simulink model "DataType"  (R2021b)
settings: Solver=VariableStepAuto  StartTime=0.0  StopTime=10.0  RelTol=1e-3
undefined symbols (not defined in the file): DiscIntNeverNeededParam, magnitude, Newton, Raphson
libraries: simulink x4, slpidlib x1
settings Model: Creator=user  LastModifiedBy=cemery

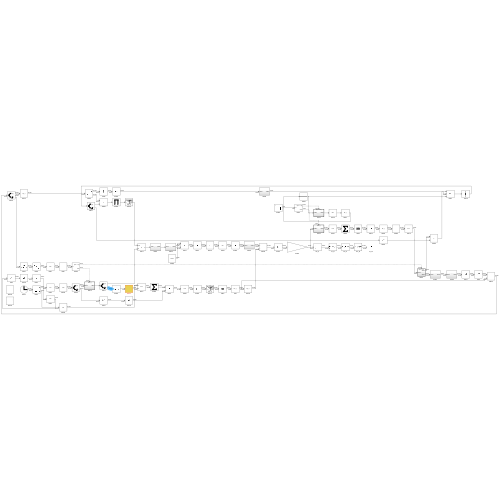
[thumbnail: Simulink's stored preview of the top-level diagram]
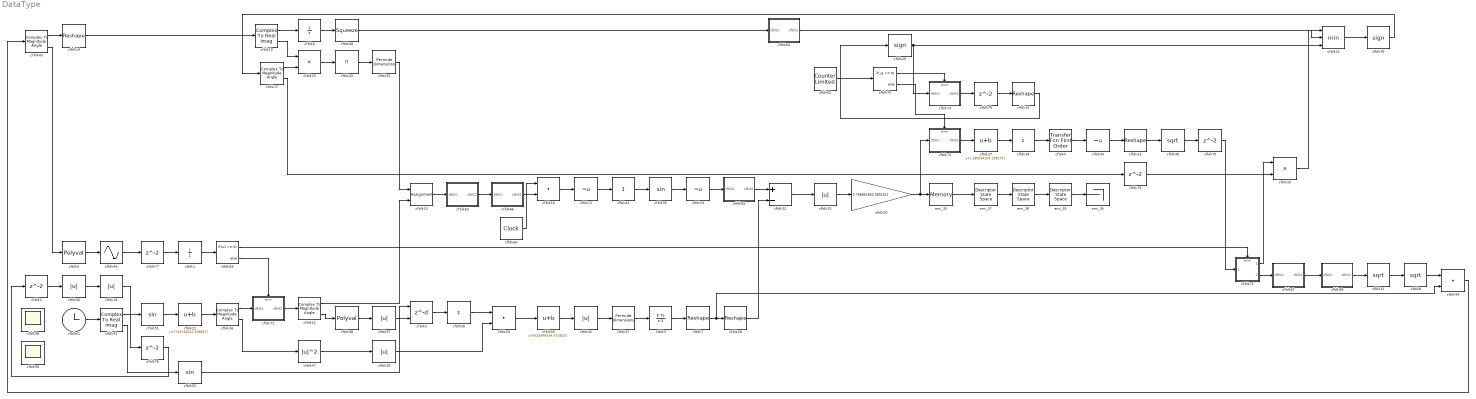
== system DataType ==
  cfblk1 : UnitDelay  HasFrameUpgradeWarning=on
  cfblk{10,18,30,42,56..57} (6 alike) : Abs
  cfblk11 : UnaryMinus
  cfblk{12,17,36,43} (4 alike) : ComplexToMagnitudeAngle
  cfblk13 : Assignment  DiagnosticForDimensions=Warning  IndexOptions=Index vector (dialog)  Indices=1  OutputSizes=1
  cfblk{7,14..15,23,28} (5 alike) : Reshape
  cfblk16 : DotProduct  InputSameDT=on  OutDataTypeStr=Inherit: Inherit via internal rule
  cfblk19 : ComplexToRealImag
  cfblk{2,75..79} (6 alike) : Delay  SampleTime=1
  cfblk20 : Gain  Gain=[-758951851.585151]
  cfblk21 : MinMax  Inputs=3
  cfblk22 : Bias  Bias=[749742041.378697]
  cfblk24 : simulink/Math Operations/Slider Gain  gain=1  low=0  high=2
  cfblk25 : Product
  cfblk26 : Sum  Inputs=+
  cfblk27 : Bias  Bias=[-185034104.199175]
  cfblk29 : Signum
  cfblk3 : Delay  DelayLengthSource=Input port  SampleTime=1
      settings: InputPortMap=u0,p1
  cfblk31 : Sqrt  SaturateOnIntegerOverflow=on
  cfblk32 : Sum  Inputs=+-
  cfblk33 : Product
  cfblk34 : UnaryMinus
  cfblk35 : Trigonometry
  cfblk37 : PermuteDimensions
  cfblk38 : Polyval  Coefs=[ +2.081618890e-019, -1.441693666e-014, +4.719686976e-010, -8.536869453e-006, +1.621573104e-001, -8.087801117e+001 ]
  cfblk39 : Sum  Inputs=+
  cfblk4 : simulink/Discrete/Transfer Fcn First Order  PoleZ=0.95  ICPrevOutput=0.0  DoSatur=off
  cfblk40 : Sqrt  SaturateOnIntegerOverflow=on
  cfblk41 : ComplexToRealImag
  cfblk44 : DotProduct  InputSameDT=on  OutDataTypeStr=Inherit: Inherit via internal rule
  cfblk45 : Product  Inputs=*
  cfblk46 : Sin  TimeSource=Use external signal  SampleTime=0
  cfblk47 : Math  Operator=magnitude^2  SaturateOnIntegerOverflow=on
  cfblk48 : Squeeze
  cfblk49 : Signum
  cfblk5 : DiscreteIntegrator  ICPrevOutput=DiscIntNeverNeededParam  ICPrevScaledInput=DiscIntNeverNeededParam
  cfblk50 : Bias  Bias=[622648534.571803]
  cfblk51 : Trigonometry
  cfblk52 : PermuteDimensions
  cfblk53 : DotProduct  InputSameDT=on  OutDataTypeStr=Inherit: Inherit via internal rule
  cfblk54 : UnaryMinus
  cfblk55 : Trigonometry
  cfblk58 : Scope
      settings: Floating=on
  cfblk59 : Scope
      settings: Floating=on
  cfblk6 : UnitDelay  HasFrameUpgradeWarning=on
  cfblk60 : DigitalClock
  cfblk61 : Clock
  cfblk62 : simulink/Sources/Counter Limited  uplimit=[209.000000]  tsamp=-1
  cfblk63 : Subsystem
  cfblk64 : Subsystem
  cfblk65 : Subsystem
  cfblk66 : Subsystem
  cfblk67 : Subsystem
  cfblk68 : Subsystem
  cfblk69 : If  IfExpression=u1 >= 0  SampleTime=1
  cfblk70 : If  IfExpression=u1 >= 0  SampleTime=1
  cfblk71 : Subsystem  TreatAsAtomicUnit=on
  cfblk72 : Subsystem  TreatAsAtomicUnit=on
  cfblk73 : Subsystem  TreatAsAtomicUnit=on
  cfblk74 : Subsystem  TreatAsAtomicUnit=on
  cfblk8 : Sqrt  SaturateOnIntegerOverflow=on
  cfblk9 : Polyval  Coefs=[ +2.081618890e-019, -1.441693666e-014, +4.719686976e-010, -8.536869453e-006, +1.621573104e-001, -8.087801117e+001 ]
  emi_35 : Memory
  emi_36 : Terminator
  emi_37 : DescriptorStateSpace
  emi_38 : DescriptorStateSpace
  emi_39 : DescriptorStateSpace
  wires:
  cfblk38/1 -> cfblk57/1
  cfblk52/1 -> cfblk13/1
  cfblk28/1 -> cfblk32/2
  cfblk74/1(cfblk2) -> cfblk27/1
  cfblk18/1 -> cfblk78/1
  cfblk73/1(cfblk2) -> cfblk79/1
  cfblk30/1 -> cfblk53/2
  cfblk70/2 -> cfblk74/Action
  emi_39/1 -> emi_36/1
  cfblk78/1 -> cfblk2/1
  cfblk26/1 -> cfblk53/1
  cfblk41/2 -> cfblk55/1
  cfblk61/1 -> cfblk41/1
  emi_38/1 -> emi_39/1
  cfblk1/1 -> cfblk69/1
  emi_37/1 -> emi_38/1
  cfblk19/2 -> cfblk25/1
  cfblk55/1 -> cfblk3/1
  cfblk46/1 -> cfblk77/1
  emi_35/1 -> emi_37/1
  cfblk9/1 -> cfblk46/1
  cfblk37/1 -> cfblk5/1
  cfblk12/2 -> cfblk38/1
  cfblk79/1 -> cfblk15/1
  cfblk77/1 -> cfblk1/1
  cfblk6/1 -> cfblk48/1
  cfblk4/1 -> cfblk34/1
  cfblk47/1 -> cfblk30/1
  cfblk76/1 -> cfblk33/2
  cfblk67/1(cfblk2) -> cfblk68/1(cfblk1)
  cfblk17/2 -> cfblk76/1
  cfblk49/1 -> cfblk17/1
  cfblk54/1 -> cfblk65/1(cfblk1)
  cfblk75/1 -> cfblk71/1(cfblk1)
  cfblk40/1 -> cfblk75/1
  cfblk25/1 -> cfblk45/1
  cfblk70/1 -> cfblk73/Action
  cfblk57/1 -> cfblk3/2
  cfblk69/2 -> cfblk72/Action
  cfblk69/1 -> cfblk71/Action
  cfblk19/1 -> cfblk6/1
  cfblk64/1(cfblk2) -> cfblk21/2
  cfblk51/1 -> cfblk22/1
  cfblk17/1 -> cfblk25/2
  cfblk71/1(cfblk2) -> cfblk33/1
  cfblk62/1 -> cfblk70/1
  cfblk32/1 -> cfblk10/1
  cfblk22/1 -> cfblk36/1
  cfblk21/1 -> cfblk49/1
  cfblk71/2(cfblk4) -> cfblk67/1(cfblk1)
  cfblk33/1 -> cfblk21/1
  cfblk2/1 -> cfblk56/1
  cfblk68/1(cfblk2) -> cfblk31/1
  cfblk36/2 -> cfblk47/1
  cfblk12/1 -> cfblk13/2
  cfblk14/1 -> cfblk19/1
  cfblk50/1 -> cfblk42/1
  cfblk66/1(cfblk2) -> cfblk16/2
  cfblk36/1 -> cfblk72/1(cfblk1)
  cfblk3/1 -> cfblk26/1
  cfblk16/1 -> cfblk11/1
  cfblk53/1 -> cfblk50/1
  cfblk41/1 -> cfblk51/1
  cfblk45/1 -> cfblk52/1
  cfblk27/1 -> cfblk39/1
  cfblk60/1 -> cfblk16/1
  cfblk15/1 -> cfblk29/1
  cfblk10/1 -> cfblk20/1
  cfblk11/1 -> cfblk24/1
  cfblk44/1 -> cfblk43/1
  cfblk34/1 -> cfblk23/1
  cfblk8/1 -> cfblk44/1
  cfblk63/1(cfblk2) -> cfblk66/1(cfblk1)
  cfblk48/1 -> cfblk64/1(cfblk1)
  cfblk65/1(cfblk2) -> cfblk32/1
  cfblk31/1 -> cfblk8/1
  cfblk35/1 -> cfblk54/1
  cfblk24/1 -> cfblk35/1
  cfblk43/2 -> cfblk9/1
  cfblk72/1(cfblk2) -> cfblk12/1
  cfblk23/1 -> cfblk40/1
  cfblk13/1 -> cfblk63/1(cfblk1)
  cfblk42/1 -> cfblk37/1
  cfblk39/1 -> cfblk4/1
  cfblk43/1 -> cfblk14/1
  cfblk56/1 -> cfblk18/1
  cfblk5/1 -> cfblk7/1
  cfblk20/1 -> emi_35/1, cfblk74/1(cfblk1)
  cfblk7/1 -> cfblk28/1, cfblk44/2
  cfblk29/1 -> cfblk73/1(cfblk1), cfblk21/3

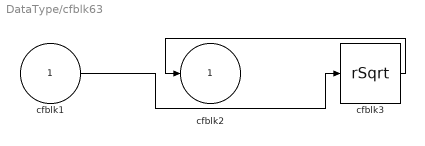
== system DataType/cfblk63 ==
  cfblk1 : Inport
  cfblk3 : Sqrt  Operator=rSqrt  AlgorithmType=Newton-Raphson  SaturateOnIntegerOverflow=on
  cfblk2 : Outport
  wires:
  cfblk3/1 -> cfblk2/1
  cfblk1/1 -> cfblk3/1

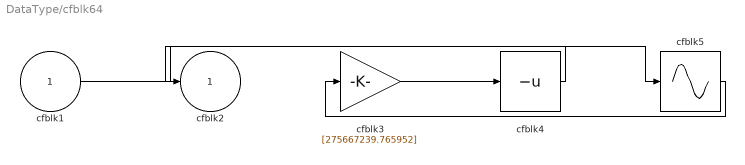
== system DataType/cfblk64 ==
  cfblk1 : Inport
  cfblk3 : Gain  Gain=[275667239.765952]
  cfblk4 : UnaryMinus
  cfblk5 : Sin  TimeSource=Use external signal  SampleTime=0
  cfblk2 : Outport
  wires:
  cfblk1/1 -> cfblk5/1
  cfblk3/1 -> cfblk4/1
  cfblk5/1 -> cfblk3/1
  cfblk4/1 -> cfblk2/1

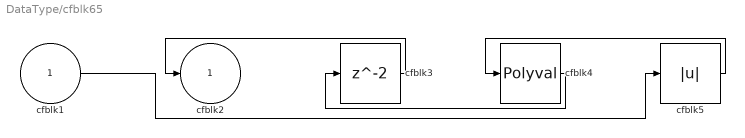
== system DataType/cfblk65 ==
  cfblk1 : Inport
  cfblk3 : Delay  SampleTime=1
  cfblk4 : Polyval  Coefs=[ +2.081618890e-019, -1.441693666e-014, +4.719686976e-010, -8.536869453e-006, +1.621573104e-001, -8.087801117e+001 ]
  cfblk5 : Abs
  cfblk2 : Outport
  wires:
  cfblk3/1 -> cfblk2/1
  cfblk5/1 -> cfblk4/1
  cfblk4/1 -> cfblk3/1
  cfblk1/1 -> cfblk5/1

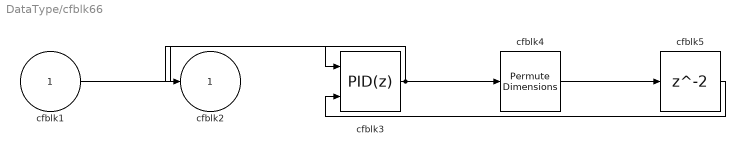
== system DataType/cfblk66 ==
  cfblk1 : Inport
  cfblk3 : slpidlib/PID Controller (2DOF)  Controller=PID  Form=Parallel  TimeDomain=Discrete-time  UseExternalTs=off  SampleTime=1  IntegratorMethod=Forward Euler  FilterMethod=Forward Euler  ControllerParametersSource=internal  P=1  I=1  D=0  UseFilter=on  N=100  b=1  c=1  TunerSelectOption=Transfer Function Based (PID Tuner App)  InitialConditionSource=internal  InitialConditionForIntegrator=0  InitialConditionForFilter=0  DifferentiatorICPrevScaledInput=0  ExternalReset=none  TrackingMode=off  Kt=1  LimitOutput=off  SatLimitsSource=internal  UpperSaturationLimit=inf  LowerSaturationLimit=-inf  LinearizeAsGain=off  AntiWindupMode=none  Kb=1  POutMin=[]  POutMax=[]  IOutMin=[]  IOutMax=[]  DOutMin=[]  DOutMax=[]  NOutMin=[]  NOutMax=[]  bOutMin=[]  bOutMax=[]  cOutMin=[]  cOutMax=[]  SumOutMin=[]  SumOutMax=[]  SaturationOutMin=[]  SaturationOutMax=[]  PParamMin=[]  PParamMax=[]  IParamMin=[]  IParamMax=[]  DParamMin=[]  DParamMax=[]  NParamMin=[]  NParamMax=[]  bParamMin=[]  bParamMax=[]  cParamMin=[]  cParamMax=[]  KbParamMin=[]  KbParamMax=[]  KtParamMin=[]  KtParamMax=[]  KbOutMin=[]  KbOutMax=[]  KtOutMin=[]  KtOutMax=[]  IntegratorOutMin=[]  IntegratorOutMax=[]  FilterOutMin=[]  FilterOutMax=[]  SumI1OutMin=[]  SumI1OutMax=[]  SumI2OutMin=[]  SumI2OutMax=[]  SumI3OutMin=[]  SumI3OutMax=[]  SumI4OutMin=[]  SumI4OutMax=[]  SumDOutMin=[]  SumDOutMax=[]  Sum1OutMin=[]  Sum1OutMax=[]  Sum2OutMin=[]  Sum2OutMax=[]  Sum3OutMin=[]  Sum3OutMax=[]  DifferentiatorOutMin=[]  DifferentiatorOutMax=[]  FilterDiffOutCoefMin=[]  FilterDiffOutCoefMax=[]  ReciprocalOutMin=[]  ReciprocalOutMax=[]  SumDenOutMin=[]  SumDenOutMax=[]  SumNumOutMin=[]  SumNumOutMax=[]  DivideOutMin=[]  DivideOutMax=[]  UdiffTsProdOutMin=[]  UdiffTsProdOutMax=[]  NTsProdOutMin=[]  NTsProdOutMax=[]  UintegralTsProdOutMin=[]  UintegralTsProdOutMax=[]  UngainTsProdOutMin=[]  UngainTsProdOutMax=[]  IntegratorContinuousStateAttributes=''  IntegratorStateMustResolveToSignalObject=off  IntegratorRTWStateStorageClass=Auto  FilterContinuousStateAttributes=''  FilterStateMustResolveToSignalObject=off  FilterRTWStateStorageClass=Auto  ParallelPVariant=InternalParameters  IdealPVariant=Disabled  IVariant=InternalParameters  DVariant=InternalParameters  bVariant=InternalParameters  cVariant=InternalParameters  IntegratorVariant=Discrete  SatVariant=Disabled  AWVariant=Passthrough  PCopyVariant=Disabled  TRVariant=Disabled  FdbkBlocksVariant=Forward  IdealPFdbkVariant=Disabled  SatFdbkVariant=Disabled  DerivativeFilterVariant=ForwardEulerFilter  NVariant=InternalParameters  NCopyVariant=Disabled  FilterICVariant=InternalICsFilter  IntegratorICVariant=InternalICs  ExternalResetVariant=Disabled  TRSumVariant=Passthrough  SumFdbkVariant=Disabled  SumVariant=Sum_PID  TsampFilterVariant=InternalTs  TsampNgainVariant=Passthrough  TsampIntegralVariant=Passthrough  ExternalSaturationOutDataTypeStr=Inherit: Same as second input
      settings: SourceProductBaseCode=SL
  cfblk4 : PermuteDimensions
  cfblk5 : Delay  SampleTime=1
  cfblk2 : Outport
  wires:
  cfblk3/1 -> cfblk4/1, cfblk2/1
  cfblk1/1 -> cfblk3/1
  cfblk4/1 -> cfblk5/1
  cfblk5/1 -> cfblk3/2

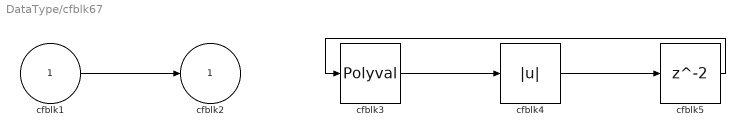
== system DataType/cfblk67 ==
  cfblk1 : Inport
  cfblk3 : Polyval  Coefs=[ +2.081618890e-019, -1.441693666e-014, +4.719686976e-010, -8.536869453e-006, +1.621573104e-001, -8.087801117e+001 ]
  cfblk4 : Abs
  cfblk5 : Delay  SampleTime=1
  cfblk2 : Outport
  wires:
  cfblk1/1 -> cfblk2/1
  cfblk3/1 -> cfblk4/1
  cfblk4/1 -> cfblk5/1
  cfblk5/1 -> cfblk3/1

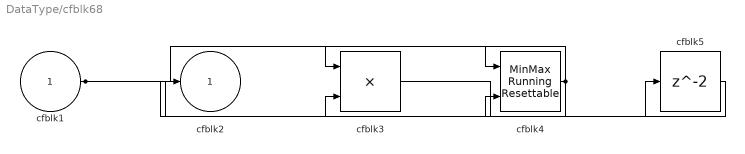
== system DataType/cfblk68 ==
  cfblk1 : Inport
  cfblk3 : Product
  cfblk4 : simulink/Math Operations/MinMax Running Resettable  Function=min  vinit=0.0
  cfblk5 : Delay  SampleTime=1
  cfblk2 : Outport
  wires:
  cfblk1/1 -> cfblk4/1, cfblk3/2
  cfblk4/1 -> cfblk2/1, cfblk3/1
  cfblk3/1 -> cfblk5/1
  cfblk5/1 -> cfblk4/2

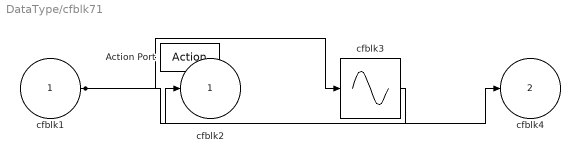
== system DataType/cfblk71 ==
  cfblk1 : Inport
  Action Port : ActionPort  ActionPortLabel=if(u1 >= 0)
  cfblk3 : Sin  TimeSource=Use external signal  SampleTime=0
  cfblk2 : Outport
  cfblk4 : Outport  Port=2
  wires:
  cfblk3/1 -> cfblk2/1
  cfblk1/1 -> cfblk3/1, cfblk4/1

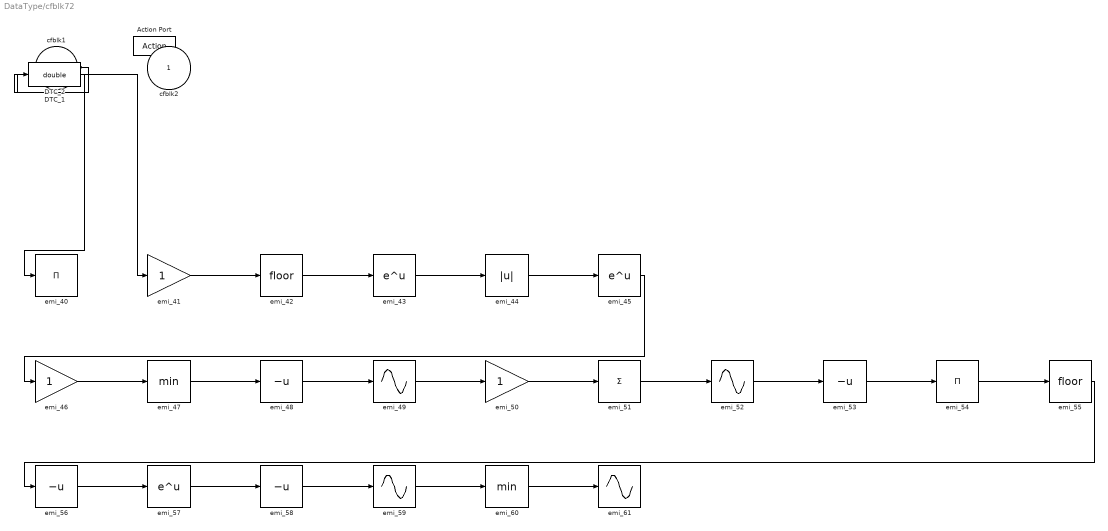
== system DataType/cfblk72 ==
  cfblk1 : Inport
  Action Port : ActionPort  ActionPortLabel=else
  DTC_1 : DataTypeConversion  OutDataTypeStr=double
  DTC_2 : DataTypeConversion  OutDataTypeStr=double
  emi_40 : Product  Inputs=*
  emi_41 : Gain
  emi_42 : Rounding
  emi_43 : Math  SaturateOnIntegerOverflow=on
  emi_44 : Abs
  emi_45 : Math  SaturateOnIntegerOverflow=on
  emi_46 : Gain
  emi_47 : MinMax
  emi_{48,53,56,58} (4 alike) : UnaryMinus
  emi_{49,52,59,61} (4 alike) : Sin  TimeSource=Use external signal  SampleTime=0
  emi_50 : Gain
  emi_51 : Sum  Inputs=+
  emi_54 : Product  Inputs=*
  emi_55 : Rounding
  emi_57 : Math  SaturateOnIntegerOverflow=on
  emi_60 : MinMax
  cfblk2 : Outport
  wires:
  cfblk1/1 -> DTC_1/1, DTC_2/1
  DTC_1/1 -> emi_40/1
  DTC_2/1 -> emi_41/1
  emi_41/1 -> emi_42/1
  emi_42/1 -> emi_43/1
  emi_43/1 -> emi_44/1
  emi_44/1 -> emi_45/1
  emi_45/1 -> emi_46/1
  emi_46/1 -> emi_47/1
  emi_47/1 -> emi_48/1
  emi_48/1 -> emi_49/1
  emi_49/1 -> emi_50/1
  emi_50/1 -> emi_51/1
  emi_51/1 -> emi_52/1
  emi_52/1 -> emi_53/1
  emi_53/1 -> emi_54/1
  emi_54/1 -> emi_55/1
  emi_55/1 -> emi_56/1
  emi_56/1 -> emi_57/1
  emi_57/1 -> emi_58/1
  emi_58/1 -> emi_59/1
  emi_59/1 -> emi_60/1
  emi_60/1 -> emi_61/1

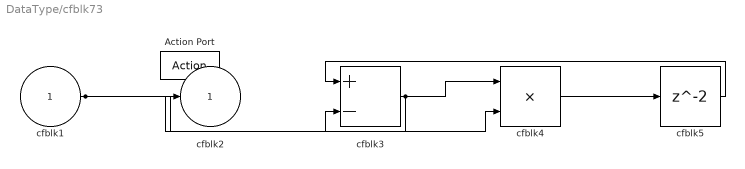
== system DataType/cfblk73 ==
  cfblk1 : Inport
  Action Port : ActionPort  ActionPortLabel=if(u1 >= 0)
  cfblk3 : Sum  Inputs=+-
  cfblk4 : Product  Inputs=**
  cfblk5 : Delay
  cfblk2 : Outport
  wires:
  cfblk3/1 -> cfblk4/1, cfblk2/1
  cfblk1/1 -> cfblk3/2, cfblk4/2
  cfblk4/1 -> cfblk5/1
  cfblk5/1 -> cfblk3/1

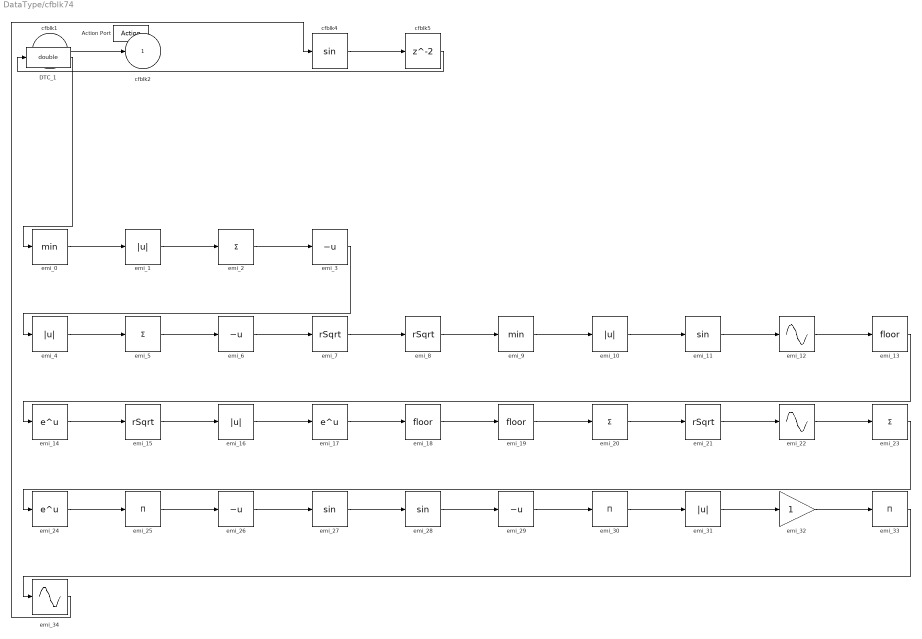
== system DataType/cfblk74 ==
  cfblk1 : Inport
  Action Port : ActionPort  ActionPortLabel=else
  DTC_1 : DataTypeConversion  OutDataTypeStr=double
  cfblk4 : Trigonometry
  cfblk5 : Delay
  emi_0 : MinMax
  emi_{1,4,10,16,31} (5 alike) : Abs
  emi_11 : Trigonometry
  emi_12 : Sin  TimeSource=Use external signal  SampleTime=0
  emi_13 : Rounding
  emi_14 : Math  SaturateOnIntegerOverflow=on
  emi_{7..8,15,21} (4 alike) : Sqrt  Operator=rSqrt  SaturateOnIntegerOverflow=on
  emi_17 : Math  SaturateOnIntegerOverflow=on
  emi_18 : Rounding
  emi_19 : Rounding
  emi_{2,5,20,23} (4 alike) : Sum  Inputs=+
  emi_22 : Sin  TimeSource=Use external signal  SampleTime=0
  emi_24 : Math  SaturateOnIntegerOverflow=on
  emi_25 : Product  Inputs=*
  emi_{3,6,26,29} (4 alike) : UnaryMinus
  emi_27 : Trigonometry
  emi_28 : Trigonometry
  emi_30 : Product  Inputs=*
  emi_32 : Gain
  emi_33 : Product  Inputs=*
  emi_34 : Sin  TimeSource=Use external signal  SampleTime=0
  emi_9 : MinMax
  cfblk2 : Outport
  wires:
  cfblk1/1 -> cfblk2/1
  cfblk4/1 -> cfblk5/1
  cfblk5/1 -> DTC_1/1
  DTC_1/1 -> emi_0/1
  emi_0/1 -> emi_1/1
  emi_1/1 -> emi_2/1
  emi_2/1 -> emi_3/1
  emi_3/1 -> emi_4/1
  emi_4/1 -> emi_5/1
  emi_5/1 -> emi_6/1
  emi_6/1 -> emi_7/1
  emi_7/1 -> emi_8/1
  emi_8/1 -> emi_9/1
  emi_9/1 -> emi_10/1
  emi_10/1 -> emi_11/1
  emi_11/1 -> emi_12/1
  emi_12/1 -> emi_13/1
  emi_13/1 -> emi_14/1
  emi_14/1 -> emi_15/1
  emi_15/1 -> emi_16/1
  emi_16/1 -> emi_17/1
  emi_17/1 -> emi_18/1
  emi_18/1 -> emi_19/1
  emi_19/1 -> emi_20/1
  emi_20/1 -> emi_21/1
  emi_21/1 -> emi_22/1
  emi_22/1 -> emi_23/1
  emi_23/1 -> emi_24/1
  emi_24/1 -> emi_25/1
  emi_25/1 -> emi_26/1
  emi_26/1 -> emi_27/1
  emi_27/1 -> emi_28/1
  emi_28/1 -> emi_29/1
  emi_29/1 -> emi_30/1
  emi_30/1 -> emi_31/1
  emi_31/1 -> emi_32/1
  emi_32/1 -> emi_33/1
  emi_33/1 -> emi_34/1
  emi_34/1 -> cfblk4/1
